simulink model "vertical_smm_3d_with_xz_lqr"  (R2015a)
settings: Solver=FixedStepDiscrete  SolverMode=SingleTasking  StartTime=0.0  StopTime=inf  FixedStep=sample_time  RelTol=1e-3
values from neighbouring files (symbols this model uses):
  forward_dx_of_dxstar = [-1.33773437568 -1.28773437515 -1.23773437461 -1.18773437408 -1.13773437355 -1.08773437301 -1.03773437248 -0.987734371946 -0.937734371413 -0.887734370879 -0.837734370532 -0.787734370254 ... (27552 elements, 41x21x32)]    [ref_trajs.mat]
  forward_x_of_dxstar = [0.243075305346 0.235858801492 0.228642297639 0.221425793786 0.214209289933 0.206992786079 0.199776282226 0.192559778373 0.18534327452 0.178126770666 0.17091026684 0.163693763058 ... (27552 elements, 41x21x32)]    [ref_trajs.mat]
  target_dx_range = [-1 -0.95 -0.9 -0.85 -0.8 -0.75 -0.7 -0.65 -0.6 -0.55 -0.5 -0.45 ... (41 elements, 1x41)]    [ref_trajs.mat]
undefined symbols (not defined in the file or in its folder): A1_notch_f1, A2_notch_f1, A_kalman_fourbar_gear, A_kalman_swing_load, A_kalman_transverse, A_kalman_vertical, A_lpf_accelerometer, A_lpf_dtau, A_lpf_fourbar_angles, A_lpf_imu, A_lpf_lateral_angle, B1_lpf_accelerometer, B1_lpf_dtau, B1_lpf_fourbar_angles, B1_lpf_imu, B1_lpf_lateral_angle, B1_notch_f1, B2_lpf_accelerometer, B2_lpf_dtau, B2_lpf_fourbar_angles, B2_lpf_imu, B2_lpf_lateral_angle, B2_notch_f1, B_dx_versus_x0, B_kalman_fourbar_gear, B_kalman_swing_load, B_kalman_transverse, B_kalman_vertical, backwards_K_sag_of_t, backwards_P_sag_of_t, C_kalman_fourbar_gear, C_kalman_swing_load, C_kalman_transverse, C_kalman_vertical, com_leg_motor, com_torso, contact_threshold, control_start_time, d_ankle_to_foot, d_vertical_com, desired_com_forward_velocity, desired_com_lateral_velocity, desired_initial_leg_roll_left, desired_initial_leg_roll_right, desired_stance_beta2, desired_standing_torso_pitch, desired_standing_torso_roll, desired_standing_z, desired_torso_pitch, desired_torso_roll, Discrete, enable_bouncing, fcut_contact, fdesignblkfcn, g, gcbh, HIP_MTR_MAX_CONT_TORQUE, HIP_MTR_MAX_TORQUE, i_leg_motor, i_robot ... (+91)
libraries: simulink x33, ctrlSharedLib x11, dsparch4 x10, dspfdesign x2
(part 4 of 7)

== system vertical_smm_3d_with_xz_lqr/Control/Behavior Control/Secondary Leg Behavior ==
  note: Convert to
      | four-bar angles
  note: Position control the
      | individual four bar segments
  note: Mirror the primary
      | leg motion
  Secondary Back Load [rad rad/s] : Inport
  Secondary Front Load [rad rad/s] : Inport  Port=2
  Torso Pitch [rad rad/s] : Inport  Port=3
  Primary Leg Angle [rad rad/s] : Inport  Port=4
  Primary Leg Length [m m/s] : Inport  Port=5
  Avoid Hitting Mechanical Limits : MATLAB Function  TreatAsAtomicUnit=on
  Back/Front PD : Subsystem
  Constant4 : Constant  Value=0
  Demux{1..3,5} (4 alike) : Demux  Outputs=2
  Demux6 : Demux  Outputs=6
  Fcn2 : Fcn  Expr=2*pi-u(1)
  Lowpass Filter (Swing) : Subsystem  DialogController=fdesignblkfcn  InitFcn=fdesignblkfcn(gcbh, {'InitFcn'});  mask(Lowpass Filter){}
      mask help: Design a lowpass filter
      settings: CopyFcn=fdesignblkfcn(gcbh, {'CopyFcn'});
      mask Help: helpview(mapfilelocation('dsp'), 'dsplowpassfilter');
      mask Display: disp('Lowpass')
  Mirrored Leg Length Target : MATLAB Function  TreatAsAtomicUnit=on
  Mux{1..4,7,11} (6 alike) : Mux  Inputs=2
  Mux5 : Mux  Inputs=3
  Mux6 : Mux  Inputs=3
  Sum : Sum  Inputs=++|
  Terminator : Terminator
  Virtual Leg to Four Bar : MATLAB Function  TreatAsAtomicUnit=on
  k_virtual1 : Gain  Gain=2
  k_virtual6 : Gain  Gain=-1
  Secondary Back/Front Motor Torque [Nm Nm] : Outport
  wires:
  Lowpass Filter (Swing)/1(Out) -> Secondary Back/Front Motor Torque [Nm Nm]/1
  Back/Front PD/1(Commanded Velocity [rad/s] [back front]) -> Lowpass Filter (Swing)/1(In)
  Mux6/1 -> Mux7/2
  Demux5/2 -> k_virtual6/1
  Mux3/1 -> Terminator/1
  Mux5/1 -> Mux7/1
  k_virtual1/1 -> Sum/1
  Torso Pitch [rad rad/s]/1 -> k_virtual1/1
  Sum/1 -> Demux5/1
  Primary Leg Length [m m/s]/1 -> Demux1/1
  Demux1/2 -> Mirrored Leg Length Target/2(primary_dl_leg)
  Demux1/1 -> Mirrored Leg Length Target/1(primary_l_leg)
  Primary Leg Angle [rad rad/s]/1 -> Sum/2
  Mux2/1 -> Back/Front PD/2(Desired Velocity [rad/s] [back front])
  Avoid Hitting Mechanical Limits/6(ddfront_cmd) -> Mux3/2
  Avoid Hitting Mechanical Limits/5(ddback_cmd) -> Mux3/1
  Avoid Hitting Mechanical Limits/4(dfront_cmd) -> Mux2/2
  Avoid Hitting Mechanical Limits/3(dback_cmd) -> Mux2/1
  Secondary Back Load [rad rad/s]/1 -> Demux3/1
  Secondary Front Load [rad rad/s]/1 -> Demux2/1
  Demux2/1 -> Mux4/2
  Avoid Hitting Mechanical Limits/1(back_cmd) -> Mux1/1
  Avoid Hitting Mechanical Limits/2(front_cmd) -> Mux1/2
  Demux3/1 -> Mux4/1
  Demux3/2 -> Mux11/1
  Mux1/1 -> Back/Front PD/1(Desired Position [rad] [back front])
  Mux4/1 -> Back/Front PD/3(Measured Position [rad] [back front])
  Demux2/2 -> Mux11/2
  Mux11/1 -> Back/Front PD/4(Measured Velocity [rad/s] [back front])
  Demux6/6 -> Virtual Leg to Four Bar/6(ddphi)
  Demux6/5 -> Virtual Leg to Four Bar/5(dphi)
  Demux6/4 -> Virtual Leg to Four Bar/4(phi)
  Demux6/3 -> Virtual Leg to Four Bar/3(ddl_leg)
  Demux6/2 -> Virtual Leg to Four Bar/2(dl_leg)
  Demux6/1 -> Virtual Leg to Four Bar/1(l_leg)
  Virtual Leg to Four Bar/6(ddfront) -> Avoid Hitting Mechanical Limits/6(ddfront_desired)
  Virtual Leg to Four Bar/5(dfront) -> Avoid Hitting Mechanical Limits/5(dfront_desired)
  Virtual Leg to Four Bar/4(front) -> Avoid Hitting Mechanical Limits/4(front_desired)
  Virtual Leg to Four Bar/3(ddback) -> Avoid Hitting Mechanical Limits/3(ddback_desired)
  Virtual Leg to Four Bar/2(dback) -> Avoid Hitting Mechanical Limits/2(dback_desired)
  Virtual Leg to Four Bar/1(back) -> Avoid Hitting Mechanical Limits/1(back_desired)
  Mux7/1 -> Demux6/1
  Fcn2/1 -> Mux6/1
  k_virtual6/1 -> Mux6/2
  Constant4/1 -> Mux6/3
  Mirrored Leg Length Target/1(l_leg) -> Mux5/1
  Mirrored Leg Length Target/3(ddl_leg) -> Mux5/3
  Mirrored Leg Length Target/2(dl_leg) -> Mux5/2
  Demux5/1 -> Fcn2/1

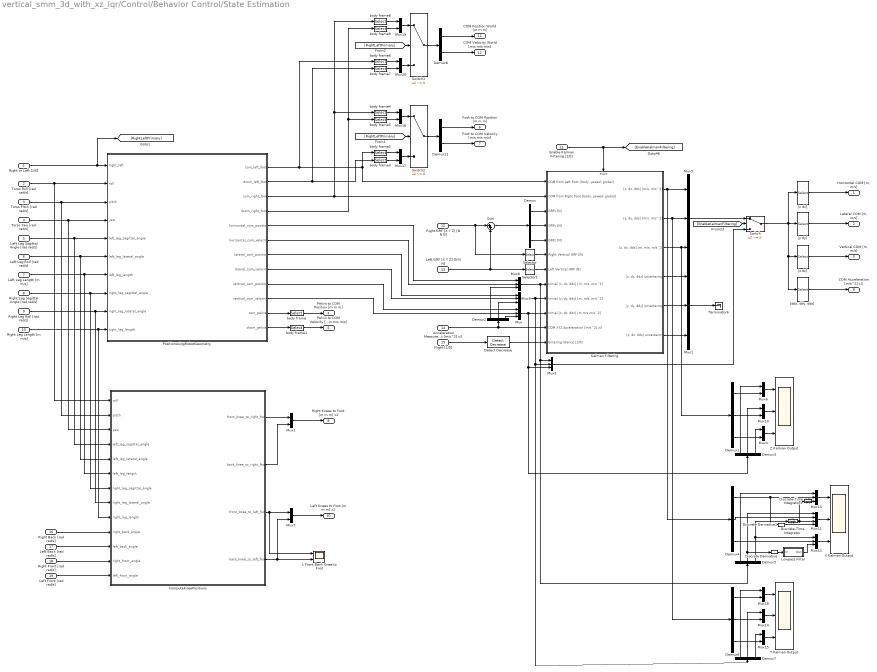
== system vertical_smm_3d_with_xz_lqr/Control/Behavior Control/State Estimation ==
  Right or Left [1/0] : Inport
  Torso Roll [rad rad/s] : Inport  Port=2
  Torso Pitch [rad rad/s] : Inport  Port=3
  Torso Yaw [rad rad/s] : Inport  Port=4
  Left Leg Sagittal Angle [rad rad/s] : Inport  Port=5
  Left Leg Roll [rad rad/s] : Inport  Port=6
  Left Leg Length [m m/s] : Inport  Port=7
  Right Leg Sagittal Angle [rad rad/s] : Inport  Port=8
  Right Leg Roll [rad rad/s] : Inport  Port=9
  Right Leg Length [m m/s] : Inport  Port=10
  Enable Kalman Filtering [1/0] : Inport  Port=11
  Right GRF [X Y Z] [N N N] : Inport  Port=12
  Left GRF [X Y Z] [N N N] : Inport  Port=13
  " Acceleration Measurement [m/s^2] x3" : Inport  Port=14
  Flight [1/0] : Inport  Port=15
  Right Back [rad rad/s] : Inport  Port=16
  Left Back [rad rad/s] : Inport  Port=17
  Right Front [rad rad/s] : Inport  Port=18
  Left Front [rad rad/s] : Inport  Port=19
  ComputeKneePositions : MATLAB Function  TreatAsAtomicUnit=on
  Demux{,1..7} (8 alike) : Demux  Outputs=3
  Demux11 : Demux  Outputs=2
  Demux8 : Demux  Outputs=2
  Detect Decrease : simulink/Logic and Bit Operations/Detect Decrease  vinit=0.0  InputProcessing=Inherited  OutDataTypeStr=boolean
  Discrete Derivative : simulink/Discrete/Discrete Derivative  gainval=1.0  ICPrevScaledInput=0.0  InputProcessing=Inherited  OutMin=[]  OutMax=[]  OutDataType=fixdt(1, 16)  OutScaling=2^-10  DoSatur=off
  Discrete Derivative1 : simulink/Discrete/Discrete Derivative  gainval=1.0  ICPrevScaledInput=0.0  InputProcessing=Inherited  OutMin=[]  OutMax=[]  OutDataType=fixdt(1, 16)  OutScaling=2^-10  DoSatur=off
  Discrete-Time Integrator : DiscreteIntegrator  InitialConditionSetting=State (most efficient)  SampleTime=-1
  Discrete-Time Integrator1 : DiscreteIntegrator  InitialConditionSetting=State (most efficient)  SampleTime=-1
  Kalman Filtering : Subsystem
  L Front Back Knee to Foot : Scope  NumInputPorts=2
      settings: YMin=-0.425~-0.5  YMax=-0.025~0.3  SaveName=ScopeData44  SampleInput=on
  Lowpass Filter : Subsystem  DialogController=fdesignblkfcn  InitFcn=fdesignblkfcn(gcbh, {'InitFcn'});  mask(Lowpass Filter){}
      mask help: Design a lowpass filter
      settings: CopyFcn=fdesignblkfcn(gcbh, {'CopyFcn'});
      mask Help: helpview(mapfilelocation('dsp'), 'dsplowpassfilter');
      mask Display: disp('Lowpass')
  Mux{,1,3,5,8..9,12..13} (8 alike) : Mux  Inputs=3
  Mux{2,4,6..7,10,14..20} (12 alike) : Mux  Inputs=2
  Mux11 : Mux
  PositionUsingRobotGeometry : MATLAB Function  TreatAsAtomicUnit=on
  Selector : Selector  InputPortWidth=3  Indices=[3]
  Selector1 : Selector  InputPortWidth=3  Indices=[3]
  Sum : Sum  Inputs=|++
  Switch : Switch  Criteria=u2 ~= 0
  Switch1 : Switch  Criteria=u2 ~= 0
  Switch2 : Switch  Criteria=u2 ~= 0
  Terminator6 : Terminator
  X Kalman Output : Scope  NumInputPorts=3
      settings: TimeRange=3.774467455621291  YMin=5.55112e-17~-0.075~-0.5  YMax=2.1~0.25~0.6  SaveName=ScopeData29  SampleInput=on
  Y Kalman Output : Scope  NumInputPorts=3
      settings: TimeRange=39.999  YMin=0.05~-0.7~-2  YMax=0.18~1.1~3.5  SaveName=ScopeData30  SampleInput=on
  Z Kalman Output : Scope  NumInputPorts=3
      settings: TimeRange=3.175000000000004  YMin=0~-0.04~-0.7  YMax=0.9~0.035~0.6  SaveName=ScopeData27  SampleInput=on
  "[ddx, ddy, ddz]" : Selector  InputPortWidth=9  Indices=[3 6 9]
  "[x dx]" : Selector  InputPortWidth=9  Indices=[1 2]
  "[y dy]" : Selector  InputPortWidth=9  Indices=[4 5]
  "[z dz]" : Selector  InputPortWidth=9  Indices=[7 8]
  body frame : Selector  InputPortWidth=9  Indices=[1 2 3]
  body frame1 : Selector  InputPortWidth=9  Indices=[1 2 3]
  body frame{2..5} (4 alike) : Selector  InputPortWidth=9  Indices=[4 5 6]
  body frame{6..9} (4 alike) : Selector  InputPortWidth=9  Indices=[7 8 9]
  "Horizontal COM [m, m/s]" : Outport
  "Lateral COM [m, m/s]" : Outport  Port=2
  "Vertical COM [m, m/s]" : Outport  Port=3
  Pelvis to COM Position [m m m] : Outport  Port=4
  Pelvis to COM Velocity [m/s m/s m/s] : Outport  Port=5
  Foot to COM Position [m m m] : Outport  Port=6
  Foot to COM Velocity [m/s m/s m/s] : Outport  Port=7
  COM Acceleration [m/s^2] x3 : Outport  Port=8
  Right Knees to Foot [m m m] x2 : Outport  Port=9
  Left Knees to Foot [m m m] x2 : Outport  Port=10
  COM Position World [m m m] : Outport  Port=11  PortDimensions=3
  COM Velocity World [m/s m/s m/s] : Outport  Port=12  PortDimensions=3
  wires:
  Discrete Derivative1/1 -> Mux11/4
  body frame8/1 -> Mux19/1
  body frame9/1 -> Mux19/2
  body frame7/1 -> Mux20/2
  body frame6/1 -> Mux20/1
  Demux8/1 -> COM Position World [m m m]/1
  Demux8/2 -> COM Velocity World [m/s m/s m/s]/1
  Switch1/1 -> Demux8/1
  Mux19/1 -> Switch1/1
  Mux20/1 -> Switch1/3
  [RightLeftPrimary] -> Switch1/2
  PositionUsingRobotGeometry/4(dcom_right_foot) -> body frame5/1, body frame9/1
  PositionUsingRobotGeometry/3(com_right_foot) -> Kalman Filtering/2("COM from Right Foot [body, yawed, global]"), body frame4/1, body frame8/1
  PositionUsingRobotGeometry/2(dcom_left_foot) -> body frame3/1, body frame7/1
  PositionUsingRobotGeometry/1(com_left_foot) -> Kalman Filtering/1("COM from Left Foot [body, yawed, global]"), body frame2/1, body frame6/1
  [EnableKalmanFiltering] -> Switch/2
  Right Back [rad rad/s]/1 -> ComputeKneePositions/10(right_back_angle)
  Left Back [rad rad/s]/1 -> ComputeKneePositions/11(left_back_angle)
  Right Front [rad rad/s]/1 -> ComputeKneePositions/12(right_front_angle)
  Left Front [rad rad/s]/1 -> ComputeKneePositions/13(left_front_angle)
  Mux7/1 -> Left Knees to Foot [m m m] x2/1
  Mux2/1 -> Right Knees to Foot [m m m] x2/1
  ComputeKneePositions/4(back_knee_to_left_foot) -> Mux7/2, L Front Back Knee to Foot/2
  ComputeKneePositions/3(front_knee_to_left_foot) -> Mux7/1, L Front Back Knee to Foot/1
  ComputeKneePositions/2(back_knee_to_right_foot) -> Mux2/2
  ComputeKneePositions/1(front_knee_to_right_foot) -> Mux2/1
  Demux7/3 -> Mux15/1
  Demux7/2 -> Mux14/1
  Demux7/1 -> Mux18/1
  Demux6/3 -> Mux15/2
  Mux14/1 -> Y Kalman Output/2
  Demux6/1 -> Mux18/2
  Demux6/2 -> Mux14/2
  Mux18/1 -> Y Kalman Output/1
  Mux15/1 -> Y Kalman Output/3
  Demux3/3 -> Mux4/1
  Demux3/2 -> Mux10/1
  Demux3/1 -> Mux6/1
  Demux1/3 -> Mux4/2
  Mux10/1 -> Z Kalman Output/2
  Demux1/1 -> Mux6/2
  Demux1/2 -> Mux10/2
  Mux6/1 -> Z Kalman Output/1
  Mux4/1 -> Z Kalman Output/3
  Detect Decrease/1 -> Kalman Filtering/12(Entering Stance [1/0])
  Flight [1/0]/1 -> Detect Decrease/1
  body frame4/1 -> Mux16/1
  body frame5/1 -> Mux16/2
  body frame3/1 -> Mux17/2
  body frame2/1 -> Mux17/1
  Demux11/1 -> Foot to COM Position [m m m]/1
  Demux11/2 -> Foot to COM Velocity [m/s m/s m/s]/1
  Switch2/1 -> Demux11/1
  Mux16/1 -> Switch2/1
  Mux17/1 -> Switch2/3
  [RightLeftPrimary] -> Switch2/2
  PositionUsingRobotGeometry/6(horizontal_com_velocity) -> Mux8/2
  PositionUsingRobotGeometry/8(lateral_com_velocity) -> Mux9/2
  Mux/1 -> Kalman Filtering/10("Initial [z, dz, ddz] [m m/s m/s^2]"), Demux3/1, Mux3/3
  PositionUsingRobotGeometry/10(vertical_com_velocity) -> Mux/2
  PositionUsingRobotGeometry/9(vertical_com_position) -> Mux/1
  Kalman Filtering/6("[z, dz, ddz] uncertainty") -> Mux1/3
  Kalman Filtering/4("[x, dx, ddx] uncertainty") -> Mux1/1
  Kalman Filtering/5("[y, dy, ddy] uncertainty") -> Mux1/2
  Kalman Filtering/2("[y, dy, ddy] [m/s, m/s^2]") -> Mux5/2, Demux6/1
  Kalman Filtering/3("[z, dz, ddz] [m, m/s, m/s^2]") -> Mux5/3, Demux1/1
  Kalman Filtering/1("[x, dx, ddx] [m/s, m/s^2]") -> Demux4/1, Mux5/1
  Demux/2 -> Kalman Filtering/4(GRFy [N])
  Demux/3 -> Kalman Filtering/5(GRFz [N])
  "[y dy]"/1 -> "Lateral COM [m, m/s]"/1
  Switch/1 -> "[ddx, ddy, ddz]"/1, "[z dz]"/1, "[y dy]"/1, "[x dx]"/1
  "[z dz]"/1 -> "Vertical COM [m, m/s]"/1
  PositionUsingRobotGeometry/7(lateral_com_position) -> Mux9/1
  body frame1/1 -> Pelvis to COM Velocity [m/s m/s m/s]/1
  body frame/1 -> Pelvis to COM Position [m m m]/1
  "[x dx]"/1 -> "Horizontal COM [m, m/s]"/1
  PositionUsingRobotGeometry/11(com_pelvis) -> body frame/1
  PositionUsingRobotGeometry/12(dcom_pelvis) -> body frame1/1
  Mux1/1 -> Terminator6/1
  Demux/1 -> Kalman Filtering/3(GRFx [N])
  Enable Kalman Filtering [1/0]/1 -> [EnableKalmanFiltering], Kalman Filtering/Enable
  Sum/1 -> Demux/1
  Right GRF [X Y Z] [N N N]/1 -> Sum/1, Selector/1
  Left GRF [X Y Z] [N N N]/1 -> Sum/2, Selector1/1
  Selector1/1 -> Kalman Filtering/7(Left Vertical GRF [N])
  Selector/1 -> Kalman Filtering/6(Right Vertical GRF [N])
  Mux5/1 -> Switch/1
  Torso Pitch [rad rad/s]/1 -> ComputeKneePositions/2(pitch), PositionUsingRobotGeometry/3(pitch)
  Torso Yaw [rad rad/s]/1 -> ComputeKneePositions/3(yaw), PositionUsingRobotGeometry/4(yaw)
  Torso Roll [rad rad/s]/1 -> ComputeKneePositions/1(roll), PositionUsingRobotGeometry/2(roll)
  Right or Left [1/0]/1 -> PositionUsingRobotGeometry/1(right_left), [RightLeftPrimary]
  Right Leg Length [m m/s]/1 -> PositionUsingRobotGeometry/10(right_leg_length), ComputeKneePositions/9(right_leg_length)
  Right Leg Roll [rad rad/s]/1 -> PositionUsingRobotGeometry/9(right_leg_lateral_angle), ComputeKneePositions/8(right_leg_lateral_angle)
  Right Leg Sagittal Angle [rad rad/s]/1 -> ComputeKneePositions/7(right_leg_sagittal_angle), PositionUsingRobotGeometry/8(right_leg_sagittal_angle)
  Left Leg Length [m m/s]/1 -> ComputeKneePositions/6(left_leg_length), PositionUsingRobotGeometry/7(left_leg_length)
  Left Leg Roll [rad rad/s]/1 -> ComputeKneePositions/5(left_leg_lateral_angle), PositionUsingRobotGeometry/6(left_leg_lateral_angle)
  Left Leg Sagittal Angle [rad rad/s]/1 -> ComputeKneePositions/4(left_leg_sagittal_angle), PositionUsingRobotGeometry/5(left_leg_sagittal_angle)
  PositionUsingRobotGeometry/5(horizontal_com_position) -> Mux8/1
  " Acceleration Measurement [m/s^2] x3"/1 -> Kalman Filtering/11(COM XYZ Acceleration [m/s^2] x3), Demux2/1
  Demux2/3 -> Mux/3
  Demux2/1 -> Mux8/3
  Demux2/2 -> Mux9/3
  Mux3/1 -> Switch/3
  "[ddx, ddy, ddz]"/1 -> COM Acceleration [m/s^2] x3/1
  Mux8/1 -> Kalman Filtering/8("Initial [x, dx, ddx] [m, m/s, m/s^2]"), Demux5/1, Mux3/1
  Mux9/1 -> Kalman Filtering/9("Initial [y, dy, ddy] [m, m/s, m/s^2]"), Demux7/1, Mux3/2
  Mux12/1 -> X Kalman Output/3
  Mux13/1 -> X Kalman Output/1
  Demux4/2 -> Mux11/2
  Demux4/1 -> Mux13/2, Discrete Derivative1/1
  Mux11/1 -> X Kalman Output/2
  Demux4/3 -> Mux12/2
  Demux5/1 -> Mux13/1
  Demux5/2 -> Discrete Derivative/1, Mux11/1
  Demux5/3 -> Discrete-Time Integrator/1, Mux12/1
  Discrete-Time Integrator/1 -> Mux11/3, Discrete-Time Integrator1/1
  Discrete Derivative/1 -> Lowpass Filter/1(In)
  Lowpass Filter/1(Out) -> Mux12/3
  Discrete-Time Integrator1/1 -> Mux13/3

== system vertical_smm_3d_with_xz_lqr/Control/Actuator Control with Torque SEA commands/Contact Velocities/Velocity on Contact ==
  in : Inport
  Trigger : TriggerPort  ShowOutputPort=on  PortDimensions=1
  Subsystem : Subsystem
  out : Outport
  wires:
  in/1 -> Subsystem/1(in)
  Subsystem/1(out) -> out/1
  Trigger/1 -> Subsystem/Enable

== system vertical_smm_3d_with_xz_lqr/Control/Actuator Control with Torque SEA commands/Contact Velocities/Velocity on Contact1 ==
  in : Inport
  Trigger : TriggerPort  ShowOutputPort=on  PortDimensions=1
  Subsystem : Subsystem
  out : Outport
  wires:
  Trigger/1 -> Subsystem/Enable
  Subsystem/1(out) -> out/1
  in/1 -> Subsystem/1(in)

== system vertical_smm_3d_with_xz_lqr/Control/Actuator Control with Torque SEA commands/Contact Velocities/Velocity on Contact2 ==
  in : Inport
  Trigger : TriggerPort  ShowOutputPort=on  PortDimensions=1
  Subsystem : Subsystem
  out : Outport
  wires:
  Trigger/1 -> Subsystem/Enable
  Subsystem/1(out) -> out/1
  in/1 -> Subsystem/1(in)

== system vertical_smm_3d_with_xz_lqr/Control/Actuator Control with Torque SEA commands/Contact Velocities/Velocity on Contact3 ==
  in : Inport
  Trigger : TriggerPort  ShowOutputPort=on  PortDimensions=1
  Subsystem : Subsystem
  out : Outport
  wires:
  in/1 -> Subsystem/1(in)
  Subsystem/1(out) -> out/1
  Trigger/1 -> Subsystem/Enable

== system vertical_smm_3d_with_xz_lqr/Control/Actuator Control with Torque SEA commands/SEA Controller (Torque)/Antiresonance Compensation ==
  Torque : Inport
  Notch Filter (Flight) : DiscreteTransferFcn  Numerator=[K_notch_f1 K_notch_f1*A1_notch_f1 K_notch_f1*A2_notch_f1]  Denominator=[1 B1_notch_f1 B2_notch_f1]  SampleTime=sample_time
  Filtered Torque : Outport
  wires:
  Torque/1 -> Notch Filter (Flight)/1
  Notch Filter (Flight)/1 -> Filtered Torque/1

== system vertical_smm_3d_with_xz_lqr/Control/Actuator Control with Torque SEA commands/SEA Controller (Torque)/Friction Compensation ==
  Motor Velocity [rad/s] : Inport
  Gain2 : Gain  Gain=sea_coulomb_friction_direction_switch_sensitivity
  KdGain2 : Gain  Description=xPCTag(1)=kd_sea_torque;  Gain=sea_coulomb_friction
  Trigonometric Function : Trigonometry  Operator=tanh
  Friction Compensation [Nm] : Outport
  wires:
  KdGain2/1 -> Friction Compensation [Nm]/1
  Motor Velocity [rad/s]/1 -> Gain2/1
  Gain2/1 -> Trigonometric Function/1
  Trigonometric Function/1 -> KdGain2/1

== system vertical_smm_3d_with_xz_lqr/Control/Actuator Control with Torque SEA commands/SEA Controller (Torque)/Loaded Unloaded Switch ==
  Loaded Signal : Inport
  Unloaded Signal : Inport  Port=2
  Loaded/Unloaded [1/0] x4 : Inport  Port=3
  Demux : Demux
  Demux1 : Demux
  Demux2 : Demux
  Mux : Mux
  Switch{,1..3} (4 alike) : Switch  Criteria=u2 ~= 0
  Signal : Outport
  wires:
  Demux/4 -> Switch3/2
  Demux/3 -> Switch2/2
  Demux/2 -> Switch1/2
  Switch1/1 -> Mux/2
  Switch2/1 -> Mux/3
  Switch3/1 -> Mux/4
  Loaded/Unloaded [1/0] x4/1 -> Demux/1
  Mux/1 -> Signal/1
  Switch/1 -> Mux/1
  Demux/1 -> Switch/2
  Loaded Signal/1 -> Demux1/1
  Demux1/1 -> Switch/1
  Demux1/2 -> Switch1/1
  Demux1/3 -> Switch2/1
  Demux1/4 -> Switch3/1
  Unloaded Signal/1 -> Demux2/1
  Demux2/4 -> Switch3/3
  Demux2/3 -> Switch2/3
  Demux2/2 -> Switch1/3
  Demux2/1 -> Switch/3

== system vertical_smm_3d_with_xz_lqr/Control/Actuator Control with Torque SEA commands/SEA Controller (Torque)/critical damping ==
  p gain : Inport
  Gain : Gain  Gain=0.75
  Gain1 : Gain  Gain=2
  Gain2 : Gain  Gain=j_motor
  Spring Stiffness1 : Gain  Gain=1./k_sea_low
  Sqrt : Sqrt  SaturateOnIntegerOverflow=on
  d gain : Outport
  wires:
  Gain1/1 -> d gain/1
  Spring Stiffness1/1 -> Gain2/1
  Gain2/1 -> Sqrt/1
  Sqrt/1 -> Gain/1
  Gain/1 -> Gain1/1
  p gain/1 -> Spring Stiffness1/1

== system vertical_smm_3d_with_xz_lqr/Control/Actuator Control with Torque SEA commands/SEA Controller (Velocity)/Integrator ==
  Signal : Inport
  Reset [1/0] : Inport  Port=2
  Demux : Demux
  Demux1 : Demux
  Discrete-Time Integrator{,1..3} (4 alike) : DiscreteIntegrator  ExternalReset=rising  InitialConditionSetting=State (most efficient)  SampleTime=sample_time  LimitOutput=on  UpperSaturationLimit=1  LowerSaturationLimit=-1
  Mux : Mux
  Integrated : Outport
  wires:
  Demux/4 -> Discrete-Time Integrator3/1
  Demux/3 -> Discrete-Time Integrator2/1
  Demux/2 -> Discrete-Time Integrator1/1
  Demux/1 -> Discrete-Time Integrator/1
  Demux1/1 -> Discrete-Time Integrator/2
  Demux1/2 -> Discrete-Time Integrator1/2
  Demux1/3 -> Discrete-Time Integrator2/2
  Demux1/4 -> Discrete-Time Integrator3/2
  Discrete-Time Integrator3/1 -> Mux/4
  Discrete-Time Integrator2/1 -> Mux/3
  Discrete-Time Integrator1/1 -> Mux/2
  Mux/1 -> Integrated/1
  Reset [1/0]/1 -> Demux1/1
  Discrete-Time Integrator/1 -> Mux/1
  Signal/1 -> Demux/1

== system vertical_smm_3d_with_xz_lqr/Control/Actuator Control with Torque SEA commands/SEA Controller (Velocity)/Lowpass Filter (Stance) ==
  In : Inport
  Generated Filter Block : DiscreteFir  Tag=BlockMethodSubSystem  Coefficients=[-0.049792265798371309 -0.00478204397482343 -0.0023545966524627579 0.0019617877955006649 0.0081617445920188422 0.01606136498204886 0.025426522925330174 0.035808512742994333 0.046780148761454213 0.057713212050140641 0.068077289761393753 0.077169075575072327 0.084565882051693325 0.089692876147162801 0.092473878579640248 0.092473878579640248 0.089692876147162801 0.084565882051693325 0.077169075575072327 0.068077289761393753 0.057713212050140641 0.046780148761454213 0.035808512742994333 0.025426522925330174 0.01606136498204886 0.0081617445920188422 0.0019617877955006649 -0.0023545966524627579 -0.00478204397482343 -0.049792265798371309]
  Out : Outport
  wires:
  Generated Filter Block/1 -> Out/1
  In/1 -> Generated Filter Block/1

== system vertical_smm_3d_with_xz_lqr/Control/Actuator Control with Torque SEA commands/SEA Controller (Velocity)/Lowpass Filter (Swing) ==
  In : Inport
  Generated Filter Block : dsparch4/Biquad Filter  Tag=BlockMethodSubSystem  IIRFiltStruct=Direct form II  CoeffSource=Specify via dialog  BiQuadCoeffs=[1.0218648663828083 -2 1.0218648663828083 1 -1.9114378222117407 0.91557643487411833]  a0Flag=Warning  IC=0  ICnum=0  ICden=0  denAccumFracLength=30  denProdOutputFracLength=30  secondMemoryFracLength=15  roundingMode=Floor  overflowMode=off  ScaleValues=[0.0041174265739107223;22.985401576126357]  optimizeScaleValues=off  ScaleValueMode=Specify via input port (g)  scaleValueFracLength=14  FilterSource=Specify via dialog  FilterObject=Hm_biquad
  Out : Outport
  wires:
  In/1 -> Generated Filter Block/1
  Generated Filter Block/1 -> Out/1

== system vertical_smm_3d_with_xz_lqr/Control/Actuator Control with Torque SEA commands/SEA Controller (Velocity)/Stance or Swing ==
  True/False x4 : Inport
  Signal True x4 : Inport  Port=2
  Signal False x4 : Inport  Port=3
  Demux : Demux
  Demux1 : Demux
  Demux2 : Demux
  Mux : Mux
  Switch{,1..3} (4 alike) : Switch  Criteria=u2 ~= 0
  Selected x4 : Outport
  wires:
  Switch3/1 -> Mux/4
  Switch2/1 -> Mux/3
  Switch1/1 -> Mux/2
  Switch/1 -> Mux/1
  Demux1/4 -> Switch3/2
  Demux1/3 -> Switch2/2
  Demux1/2 -> Switch1/2
  Demux1/1 -> Switch/2
  Demux2/4 -> Switch3/3
  Demux2/3 -> Switch2/3
  Demux2/2 -> Switch1/3
  Demux2/1 -> Switch/3
  Demux/4 -> Switch3/1
  Demux/3 -> Switch2/1
  Demux/2 -> Switch1/1
  Demux/1 -> Switch/1
  Signal False x4/1 -> Demux2/1
  Signal True x4/1 -> Demux/1
  True/False x4/1 -> Demux1/1
  Mux/1 -> Selected x4/1

== system vertical_smm_3d_with_xz_lqr/Control/Actuator Control with Torque SEA commands/SEA Controller (Velocity)/Stance or Swing1 ==
  True/False x4 : Inport
  Signal True x4 : Inport  Port=2
  Signal False x4 : Inport  Port=3
  Demux : Demux
  Demux1 : Demux
  Demux2 : Demux
  Mux : Mux
  Switch{,1..3} (4 alike) : Switch  Criteria=u2 ~= 0
  Selected x4 : Outport
  wires:
  Mux/1 -> Selected x4/1
  True/False x4/1 -> Demux1/1
  Signal True x4/1 -> Demux/1
  Signal False x4/1 -> Demux2/1
  Demux/1 -> Switch/1
  Demux/2 -> Switch1/1
  Demux/3 -> Switch2/1
  Demux/4 -> Switch3/1
  Demux2/1 -> Switch/3
  Demux2/2 -> Switch1/3
  Demux2/3 -> Switch2/3
  Demux2/4 -> Switch3/3
  Demux1/1 -> Switch/2
  Demux1/2 -> Switch1/2
  Demux1/3 -> Switch2/2
  Demux1/4 -> Switch3/2
  Switch/1 -> Mux/1
  Switch1/1 -> Mux/2
  Switch2/1 -> Mux/3
  Switch3/1 -> Mux/4

== system vertical_smm_3d_with_xz_lqr/Control/Actuator Control with Torque SEA commands/SEA Controller (Velocity)/Stance or Swing2 ==
  True/False x4 : Inport
  Signal True x4 : Inport  Port=2
  Signal False x4 : Inport  Port=3
  Demux : Demux
  Demux1 : Demux
  Demux2 : Demux
  Mux : Mux
  Switch{,1..3} (4 alike) : Switch  Criteria=u2 ~= 0
  Selected x4 : Outport
  wires:
  Switch3/1 -> Mux/4
  Switch2/1 -> Mux/3
  Switch1/1 -> Mux/2
  Switch/1 -> Mux/1
  Demux1/4 -> Switch3/2
  Demux1/3 -> Switch2/2
  Demux1/2 -> Switch1/2
  Demux1/1 -> Switch/2
  Demux2/4 -> Switch3/3
  Demux2/3 -> Switch2/3
  Demux2/2 -> Switch1/3
  Demux2/1 -> Switch/3
  Demux/4 -> Switch3/1
  Demux/3 -> Switch2/1
  Demux/2 -> Switch1/1
  Demux/1 -> Switch/1
  Signal False x4/1 -> Demux2/1
  Signal True x4/1 -> Demux/1
  True/False x4/1 -> Demux1/1
  Mux/1 -> Selected x4/1

== system vertical_smm_3d_with_xz_lqr/Control/Actuator Control with Torque SEA commands/Timers/Time on Contact ==
  in : Inport
  Trigger : TriggerPort  ShowOutputPort=on  PortDimensions=1
  Subsystem : Subsystem
  out : Outport
  wires:
  Trigger/1 -> Subsystem/Enable
  Subsystem/1(out) -> out/1
  in/1 -> Subsystem/1(in)

== system vertical_smm_3d_with_xz_lqr/Control/Actuator Control with Torque SEA commands/Timers/Time on Contact1 ==
  in : Inport
  Trigger : TriggerPort  ShowOutputPort=on  PortDimensions=1
  Subsystem : Subsystem
  out : Outport
  wires:
  in/1 -> Subsystem/1(in)
  Subsystem/1(out) -> out/1
  Trigger/1 -> Subsystem/Enable

== system vertical_smm_3d_with_xz_lqr/Control/Actuator Control with Torque SEA commands/Timers/Time on Contact2 ==
  in : Inport
  Trigger : TriggerPort  ShowOutputPort=on  PortDimensions=1
  Subsystem : Subsystem
  out : Outport
  wires:
  in/1 -> Subsystem/1(in)
  Subsystem/1(out) -> out/1
  Trigger/1 -> Subsystem/Enable

== system vertical_smm_3d_with_xz_lqr/Control/Actuator Control with Torque SEA commands/Timers/Time on Contact3 ==
  in : Inport
  Trigger : TriggerPort  ShowOutputPort=on  PortDimensions=1
  Subsystem : Subsystem
  out : Outport
  wires:
  Trigger/1 -> Subsystem/Enable
  Subsystem/1(out) -> out/1
  in/1 -> Subsystem/1(in)

== system vertical_smm_3d_with_xz_lqr/Control/Behavior Control/Atrias Swing control/Back//Front PD1 ==
  Desired Position [rad] [back front] : Inport
  Desired Velocity [rad/s] [back front] : Inport  Port=2
  Measured Position [rad] [back front] : Inport  Port=3
  Measured Velocity [rad/s] [back front] : Inport  Port=4
  Back Tracking : Scope  NumInputPorts=2
      settings: YMin=3.725~-1  YMax=4.05~0.9  SaveName=ScopeData6  SampleInput=on
  Front Tracking : Scope  NumInputPorts=2
      settings: YMin=-1~-0.8  YMax=1~1.4  SaveName=ScopeData31  SampleInput=on
  Kp_SEA_Trajectory : Constant  Value=kp_velocity_swing_trajectory
  Mux{1..2,12..13} (4 alike) : Mux  Inputs=2
  Product1 : Product
  Selector{,1..3} (4 alike) : Selector  InputPortWidth=2  Indices=[1]
  Selector{4..7} (4 alike) : Selector  InputPortWidth=2  Indices=[2]
  Sum7 : Sum  Inputs=|+-
  Sum9 : Sum
  Commanded Velocity [rad/s] [back front] : Outport
  wires:
  Kp_SEA_Trajectory/1 -> Product1/2
  Sum9/1 -> Commanded Velocity [rad/s] [back front]/1
  Measured Velocity [rad/s] [back front]/1 -> Selector7/1, Selector3/1
  Desired Velocity [rad/s] [back front]/1 -> Selector6/1, Selector2/1, Sum9/2
  Measured Position [rad] [back front]/1 -> Selector4/1, Selector/1, Sum7/2
  Sum7/1 -> Product1/1
  Product1/1 -> Sum9/1
  Mux12/1 -> Back Tracking/2
  Mux13/1 -> Back Tracking/1
  Desired Position [rad] [back front]/1 -> Selector5/1, Selector1/1, Sum7/1
  Mux1/1 -> Front Tracking/2
  Mux2/1 -> Front Tracking/1
  Selector/1 -> Mux13/1
  Selector1/1 -> Mux13/2
  Selector2/1 -> Mux12/1
  Selector3/1 -> Mux12/2
  Selector5/1 -> Mux2/2
  Selector4/1 -> Mux2/1
  Selector6/1 -> Mux1/1
  Selector7/1 -> Mux1/2

== system vertical_smm_3d_with_xz_lqr/Control/Behavior Control/Atrias Swing control/Lowpass Filter (Swing) ==
  In : Inport
  Generated Filter Block : dsparch4/Biquad Filter  Tag=BlockMethodSubSystem  IIRFiltStruct=Direct form II  CoeffSource=Specify via dialog  BiQuadCoeffs=[1.0218648663828083 -2 1.0218648663828083 1 -1.9114378222117407 0.91557643487411833]  a0Flag=Warning  IC=0  ICnum=0  ICden=0  denAccumFracLength=30  denProdOutputFracLength=30  secondMemoryFracLength=15  roundingMode=Floor  overflowMode=off  ScaleValues=[0.0041174265739107223;22.985401576126357]  optimizeScaleValues=off  ScaleValueMode=Specify via input port (g)  scaleValueFracLength=14  FilterSource=Specify via dialog  FilterObject=Hm_biquad
  Out : Outport
  wires:
  In/1 -> Generated Filter Block/1
  Generated Filter Block/1 -> Out/1

== system vertical_smm_3d_with_xz_lqr/Control/Behavior Control/Force Estimation/Leg Force Measurements ==
  q : Inport
  Leg Width Right/Left [m m] : Inport  Port=2
  Leg Length Right/Left [m m] : Inport  Port=3
  Demux : Demux  Outputs=2
  Demux1 : Demux  Outputs=2
  Demux2 : Demux
  Divide{1..4} (4 alike) : Product  Inputs=*/
  Gain : Gain  Commented=on  Gain=k_sea_low
  Mux : Mux
  Nonlinear Spring Force : MATLAB Function  TreatAsAtomicUnit=on
  Sum{1..3,6} (4 alike) : Sum  Inputs=-+|
  Sum4 : Sum  Inputs=-|+
  Sum5 : Sum  Inputs=-|+
  Sum7 : Sum  Inputs=+|+
  Sum8 : Sum  Inputs=+|+
  backGearL : Selector  InputPortWidth=13  Indices=[6]
  backGearR : Selector  InputPortWidth=13  Indices=[2]
  backJointL : Selector  InputPortWidth=13  Indices=[5]
  backJointR : Selector  InputPortWidth=13  Indices=[1]
  frontGearL : Selector  InputPortWidth=13  Indices=[8]
  frontGearR : Selector  InputPortWidth=13  Indices=[4]
  frontJointL : Selector  InputPortWidth=13  Indices=[7]
  frontJointR : Selector  InputPortWidth=13  Indices=[3]
  Right Leg Torque [Nm] : Outport
  Left Leg Torque [Nm] : Outport  Port=2
  Right Leg Axial Force [N] : Outport  Port=3
  Left Leg Axial Force [N] : Outport  Port=4
  Right Leg Orthogonal Force [N] : Outport  Port=5
  Left Leg Orthogonal Force [N] : Outport  Port=6
  wires:
  Nonlinear Spring Force/1(tau_sea) -> Demux2/1
  Mux/1 -> Nonlinear Spring Force/1(deflections)
  Divide4/1 -> Left Leg Orthogonal Force [N]/1
  Divide3/1 -> Right Leg Orthogonal Force [N]/1
  Leg Length Right/Left [m m]/1 -> Demux1/1
  Demux1/2 -> Divide4/2
  Demux1/1 -> Divide3/2
  Sum8/1 -> Left Leg Torque [Nm]/1, Divide4/1
  Sum7/1 -> Right Leg Torque [Nm]/1, Divide3/1
  Demux2/3 -> Sum5/1, Sum8/1
  Divide2/1 -> Left Leg Axial Force [N]/1
  Divide1/1 -> Right Leg Axial Force [N]/1
  Demux/2 -> Divide2/2
  Demux/1 -> Divide1/2
  Leg Width Right/Left [m m]/1 -> Demux/1
  Sum5/1 -> Divide2/1
  Sum4/1 -> Divide1/1
  Demux2/4 -> Sum8/2, Sum5/2
  Demux2/2 -> Sum4/2, Sum7/2
  Demux2/1 -> Sum7/1, Sum4/1
  q/1 -> backJointR/1, frontJointR/1, frontGearR/1, backGearL/1, frontGearL/1, frontJointL/1, backJointL/1, backGearR/1
  backGearR/1 -> Sum6/2
  frontJointR/1 -> Sum1/1
  frontGearR/1 -> Sum1/2
  backJointR/1 -> Sum6/1
  Sum1/1 -> Mux/2
  Sum6/1 -> Mux/1
  backGearL/1 -> Sum2/2
  frontJointL/1 -> Sum3/1
  frontGearL/1 -> Sum3/2
  backJointL/1 -> Sum2/1
  Sum2/1 -> Mux/3
  Sum3/1 -> Mux/4

== system vertical_smm_3d_with_xz_lqr/Control/Behavior Control/Force Estimation/Leg Plane GRF ==
  Axial Force [N] : Inport
  Orthogonal Force [N] : Inport  Port=2
  Torso Pitch [rad] : Inport  Port=3
  Leg Angle [rad] : Inport  Port=4
  Gain : Gain  Gain=-1
  Product : Product
  Product1 : Product
  Sum : Sum  Inputs=++|
  Sum1 : Sum  Inputs=+|+
  Trigonometric Function : Trigonometry  Operator=cos
  Trigonometric Function1 : Trigonometry
  Vertical Force [N] : Outport
  wires:
  Gain/1 -> Sum1/1
  Sum/1 -> Trigonometric Function1/1, Trigonometric Function/1
  Product/1 -> Gain/1
  Trigonometric Function/1 -> Product/2
  Torso Pitch [rad]/1 -> Sum/1
  Leg Angle [rad]/1 -> Sum/2
  Axial Force [N]/1 -> Product/1
  Orthogonal Force [N]/1 -> Product1/1
  Trigonometric Function1/1 -> Product1/2
  Sum1/1 -> Vertical Force [N]/1
  Product1/1 -> Sum1/2

== system vertical_smm_3d_with_xz_lqr/Control/Behavior Control/Primary and Lateral Behavior/Circular Buffer ==
  Flight [1/0] : Inport
  Exiting Stance [1/0] : Inport  Port=2
  Hopping [1/0] : Inport  Port=3
  dX [m/s] : Inport  Port=4
  dY [m/s] : Inport  Port=5
  X Foot Correction [m] : Inport  Port=6
  Y Foot Correction [m] : Inport  Port=7
  target dX [m/s] : Inport  Port=8
  target dY [m/s] : Inport  Port=9
  Buffer : MATLAB Function  TreatAsAtomicUnit=on  SystemSampleTime=sample_time
  Buffer1 : MATLAB Function  TreatAsAtomicUnit=on  SystemSampleTime=sample_time
  Buffer2 : MATLAB Function  TreatAsAtomicUnit=on  SystemSampleTime=sample_time
  Buffer3 : MATLAB Function  TreatAsAtomicUnit=on  SystemSampleTime=sample_time
  Buffer4 : MATLAB Function  TreatAsAtomicUnit=on  SystemSampleTime=sample_time
  Buffer5 : MATLAB Function  TreatAsAtomicUnit=on  SystemSampleTime=sample_time
  Buffer6 : MATLAB Function  TreatAsAtomicUnit=on  SystemSampleTime=sample_time
  Buffer7 : MATLAB Function  TreatAsAtomicUnit=on  SystemSampleTime=sample_time
  Demux : Demux  Outputs=6
  Detect Decrease : simulink/Logic and Bit Operations/Detect Decrease  vinit=0.0  InputProcessing=Inherited  OutDataTypeStr=boolean
  Enabled on Touchdown : Subsystem  TreatAsAtomicUnit=on
  Logical Operator : Logic  AllPortsSameDT=off  OutDataTypeStr=boolean
  Mux : Mux  Inputs=6
  buffer size5 : Constant  Value=recorded_steps
  "dX Touchdown History " : Outport
  X Foot Correction History : Outport  Port=2
  dX Takeoff History : Outport  Port=3
  "dY Touchdown History " : Outport  Port=4
  Y Foot Correction History : Outport  Port=5
  dY Takeoff History : Outport  Port=6
  target dX History : Outport  Port=7
  target dY History : Outport  Port=8
  wires:
  Buffer/1(buffer) -> "dX Touchdown History "/1
  Detect Decrease/1 -> Enabled on Touchdown/Enable
  Buffer1/1(buffer) -> X Foot Correction History/1
  Buffer2/1(buffer) -> dX Takeoff History/1
  Demux/1 -> Buffer/1(data)
  Demux/3 -> Buffer1/1(data)
  X Foot Correction [m]/1 -> Mux/3
  Buffer3/1(buffer) -> "dY Touchdown History "/1
  Buffer4/1(buffer) -> Y Foot Correction History/1
  Demux/2 -> Buffer3/1(data)
  Buffer5/1(buffer) -> dY Takeoff History/1
  Y Foot Correction [m]/1 -> Mux/4
  Demux/4 -> Buffer4/1(data)
  target dX [m/s]/1 -> Mux/5
  Buffer6/1(buffer) -> target dX History/1
  Buffer7/1(buffer) -> target dY History/1
  buffer size5/1 -> Buffer2/3(buffer_size), Buffer/3(buffer_size), Buffer7/3(buffer_size), Buffer6/3(buffer_size), Buffer4/3(buffer_size), Buffer1/3(buffer_size), Buffer3/3(buffer_size), Buffer5/3(buffer_size)
  Demux/6 -> Buffer7/1(data)
  Demux/5 -> Buffer6/1(data)
  target dY [m/s]/1 -> Mux/6
  Exiting Stance [1/0]/1 -> Buffer/2(trigger), Buffer7/2(trigger), Buffer6/2(trigger), Buffer4/2(trigger), Buffer1/2(trigger), Buffer3/2(trigger), Buffer2/2(trigger), Buffer5/2(trigger)
  Hopping [1/0]/1 -> Logical Operator/1
  dY [m/s]/1 -> Buffer5/1(data), Mux/2
  dX [m/s]/1 -> Buffer2/1(data), Mux/1
  Flight [1/0]/1 -> Logical Operator/2
  Logical Operator/1 -> Detect Decrease/1
  Mux/1 -> Enabled on Touchdown/1(In)
  Enabled on Touchdown/1(Out) -> Demux/1

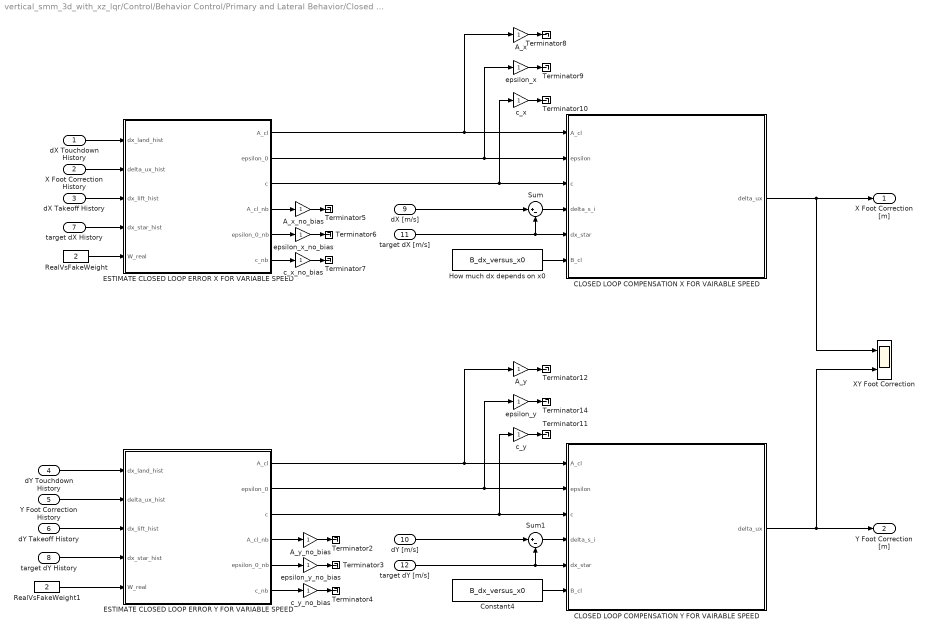
== system vertical_smm_3d_with_xz_lqr/Control/Behavior Control/Primary and Lateral Behavior/Closed Loop Compensation ==
  dX Touchdown History : Inport
  X Foot Correction History : Inport  Port=2
  dX Takeoff History : Inport  Port=3
  dY Touchdown History : Inport  Port=4
  Y Foot Correction History : Inport  Port=5
  dY Takeoff History : Inport  Port=6
  target dX History : Inport  Port=7
  target dY History : Inport  Port=8
  dX [m/s] : Inport  Port=9
  dY [m/s] : Inport  Port=10
  target dX [m/s] : Inport  Port=11
  "target dY [m/s] " : Inport  Port=12
  A_x : Gain
  A_x_no_bias : Gain
  A_y : Gain
  A_y_no_bias : Gain
  CLOSED LOOP COMPENSATION X FOR VAIRABLE SPEED : MATLAB Function  TreatAsAtomicUnit=on
  CLOSED LOOP COMPENSATION Y FOR VAIRABLE SPEED : MATLAB Function  TreatAsAtomicUnit=on
  Constant4 : Constant  Value=B_dx_versus_x0
  ESTIMATE CLOSED LOOP ERROR X FOR VARIABLE SPEED : MATLAB Function  TreatAsAtomicUnit=on
  ESTIMATE CLOSED LOOP ERROR Y FOR VARIABLE SPEED : MATLAB Function  TreatAsAtomicUnit=on
  How much dx depends on x0 : Constant  Value=B_dx_versus_x0
  RealVsFakeWeight : Constant  Value=2
  RealVsFakeWeight1 : Constant  Value=2
  Sum : Sum  Inputs=|+-
  Sum1 : Sum  Inputs=|+-
  Terminator{2..12,14} (12 alike) : Terminator
  XY Foot Correction : Scope  NumInputPorts=2
      settings: YMin=-1~-0.8  YMax=1~1.4  SaveName=ScopeData39  SampleInput=on
  c_x : Gain
  c_x_no_bias : Gain
  c_y : Gain
  c_y_no_bias : Gain
  epsilon_x : Gain
  epsilon_x_no_bias : Gain
  epsilon_y : Gain
  epsilon_y_no_bias : Gain
  X Foot Correction [m] : Outport
  Y Foot Correction [m] : Outport  Port=2
  wires:
  c_y/1 -> Terminator11/1
  epsilon_y/1 -> Terminator14/1
  A_y/1 -> Terminator12/1
  ESTIMATE CLOSED LOOP ERROR Y FOR VARIABLE SPEED/1(A_cl) -> CLOSED LOOP COMPENSATION Y FOR VAIRABLE SPEED/1(A_cl), A_y/1
  ESTIMATE CLOSED LOOP ERROR Y FOR VARIABLE SPEED/2(epsilon_0) -> CLOSED LOOP COMPENSATION Y FOR VAIRABLE SPEED/2(epsilon), epsilon_y/1
  ESTIMATE CLOSED LOOP ERROR Y FOR VARIABLE SPEED/3(c) -> CLOSED LOOP COMPENSATION Y FOR VAIRABLE SPEED/3(c), c_y/1
  c_x/1 -> Terminator10/1
  epsilon_x/1 -> Terminator9/1
  A_x/1 -> Terminator8/1
  ESTIMATE CLOSED LOOP ERROR X FOR VARIABLE SPEED/1(A_cl) -> CLOSED LOOP COMPENSATION X FOR VAIRABLE SPEED/1(A_cl), A_x/1
  ESTIMATE CLOSED LOOP ERROR X FOR VARIABLE SPEED/2(epsilon_0) -> CLOSED LOOP COMPENSATION X FOR VAIRABLE SPEED/2(epsilon), epsilon_x/1
  ESTIMATE CLOSED LOOP ERROR X FOR VARIABLE SPEED/3(c) -> CLOSED LOOP COMPENSATION X FOR VAIRABLE SPEED/3(c), c_x/1
  ESTIMATE CLOSED LOOP ERROR Y FOR VARIABLE SPEED/6(c_nb) -> c_y_no_bias/1
  ESTIMATE CLOSED LOOP ERROR Y FOR VARIABLE SPEED/5(epsilon_0_nb) -> epsilon_y_no_bias/1
  ESTIMATE CLOSED LOOP ERROR Y FOR VARIABLE SPEED/4(A_cl_nb) -> A_y_no_bias/1
  c_y_no_bias/1 -> Terminator4/1
  epsilon_y_no_bias/1 -> Terminator3/1
  A_y_no_bias/1 -> Terminator2/1
  c_x_no_bias/1 -> Terminator7/1
  epsilon_x_no_bias/1 -> Terminator6/1
  A_x_no_bias/1 -> Terminator5/1
  ESTIMATE CLOSED LOOP ERROR X FOR VARIABLE SPEED/4(A_cl_nb) -> A_x_no_bias/1
  ESTIMATE CLOSED LOOP ERROR X FOR VARIABLE SPEED/5(epsilon_0_nb) -> epsilon_x_no_bias/1
  ESTIMATE CLOSED LOOP ERROR X FOR VARIABLE SPEED/6(c_nb) -> c_x_no_bias/1
  CLOSED LOOP COMPENSATION Y FOR VAIRABLE SPEED/1(delta_ux) -> Y Foot Correction [m]/1, XY Foot Correction/2
  CLOSED LOOP COMPENSATION X FOR VAIRABLE SPEED/1(delta_ux) -> X Foot Correction [m]/1, XY Foot Correction/1
  Sum1/1 -> CLOSED LOOP COMPENSATION Y FOR VAIRABLE SPEED/4(delta_s_i)
  dY Touchdown History/1 -> ESTIMATE CLOSED LOOP ERROR Y FOR VARIABLE SPEED/1(dx_land_hist)
  dX [m/s]/1 -> Sum/1
  dX Touchdown History/1 -> ESTIMATE CLOSED LOOP ERROR X FOR VARIABLE SPEED/1(dx_land_hist)
  dX Takeoff History/1 -> ESTIMATE CLOSED LOOP ERROR X FOR VARIABLE SPEED/3(dx_lift_hist)
  X Foot Correction History/1 -> ESTIMATE CLOSED LOOP ERROR X FOR VARIABLE SPEED/2(delta_ux_hist)
  target dX History/1 -> ESTIMATE CLOSED LOOP ERROR X FOR VARIABLE SPEED/4(dx_star_hist)
  target dX [m/s]/1 -> CLOSED LOOP COMPENSATION X FOR VAIRABLE SPEED/5(dx_star), Sum/2
  Sum/1 -> CLOSED LOOP COMPENSATION X FOR VAIRABLE SPEED/4(delta_s_i)
  How much dx depends on x0/1 -> CLOSED LOOP COMPENSATION X FOR VAIRABLE SPEED/6(B_cl)
  RealVsFakeWeight/1 -> ESTIMATE CLOSED LOOP ERROR X FOR VARIABLE SPEED/5(W_real)
  dY [m/s]/1 -> Sum1/1
  dY Takeoff History/1 -> ESTIMATE CLOSED LOOP ERROR Y FOR VARIABLE SPEED/3(dx_lift_hist)
  Y Foot Correction History/1 -> ESTIMATE CLOSED LOOP ERROR Y FOR VARIABLE SPEED/2(delta_ux_hist)
  target dY History/1 -> ESTIMATE CLOSED LOOP ERROR Y FOR VARIABLE SPEED/4(dx_star_hist)
  "target dY [m/s] "/1 -> CLOSED LOOP COMPENSATION Y FOR VAIRABLE SPEED/5(dx_star), Sum1/2
  Constant4/1 -> CLOSED LOOP COMPENSATION Y FOR VAIRABLE SPEED/6(B_cl)
  RealVsFakeWeight1/1 -> ESTIMATE CLOSED LOOP ERROR Y FOR VARIABLE SPEED/5(W_real)

== system vertical_smm_3d_with_xz_lqr/Control/Behavior Control/Primary and Lateral Behavior/Enabled on Takeoff ==
  In : Inport
  Enable : EnablePort
  Out : Outport
  wires:
  In/1 -> Out/1
